simulink model "pmsm_drive"  (R2020b)
settings: Solver=VariableStepAuto  StartTime=0.0  StopTime=0.6  FixedStep=Ts  RelTol=1e-3  AbsTol=1e-3  EnableMultiTasking=on
PreLoadFcn:
  | % Control parameters
  | Ts = 2e-6;   % Fundamental sample time
  | fsw = 2e3;   % Switching frequency (Hz)
  | fc = fsw*10; % Control loop frequency (Hz)
  | Tsc = 1/fc;  % Control loop sample time
  | 
  | % PMSM parameters
  | PM = 0.03; % Permanent magnet flux linkage
  | Ld = 2e-4;  % d-axis inductance
  | Lq = 2e-4;  % q-axis inductance
  | L0 = 2e-4;  % 0-axis inductance
  | Rs = 0.013; % Stator resistance
  | N = 6; % Number of pole pairs
  | J = 0.2; % Moment of inertia
  | 
  | % Operating and derived limits
  | Imax = 100;  % Max stator current (peak value)
  | Tmax = 1.5*N*PM*Imax; % Max lectromagnetic torque
  | fnom = 100;  % Nominal frequency (Hz)
  | rpm_nom = 60*fnom/N;      % Nominal rotor speed (rpm)
  | omegam_nom = 2*pi*fnom/N; % Nominal mechanical rotor speed
  | Pmax = omegam_nom*Tmax;     % Maximum power
StopFcn:
  | ee_addSimlogTimeStamp(bdroot)
undefined symbols (not defined in the file or in its folder): ee_sli_rtmsupport, gcbh
libraries: fl_lib x10, nesl_utility x8, ee_lib x3, eeTransforms x2, eePmsmCurrentController x1, eePmsmCurrentReferenceGen x1, eeVelocityController x1, mcbplantlib x1
CloseFcn:
  | try,close(h1_ee_pmsm_drive),end
  | clear h1_ee_pmsm_drive
  | try,close(h2_ee_pmsm_drive),end
  | clear h2_ee_pmsm_drive
  | try,close(h3_ee_pmsm_drive),end
  | clear h3_ee_pmsm_drive
  | try,close(h4_ee_pmsm_drive),end
  | clear h4_ee_pmsm_drive
Description:
  | Three-Phase PMSM Drive
settings Model: Creator=The MathWorks, Inc.  LastModifiedBy=Student
settings SolverCC: AutoScaleAbsTol=off  MaxConsecutiveMinStep=2  ZeroCrossAlgorithm=Adaptive
settings DataIOCC: LimitDataPoints=on  MaxDataPoints=690000  SaveFormat=Array  ReturnWorkspaceOutputs=off  SignalLoggingName=logsout_ee_pmsm_drive
settings OptimizationCC: LifeSpan=inf
settings DebuggingCC: UnderspecifiedInitializationDetection=Classic  MergeDetectMultiDrivingBlocksExec=none  MaxConsecutiveZCsMsg=none  IgnoredZcDiagnostic=none  AllowSymbolicDim=off  PregeneratedLibrarySubsystemCodeDiagnostic=none  SFUnexpectedBacktrackingDiag=warning  SFNoUnconditionalDefaultTransitionDiag=warning  SFExecutionAtInitializationDiag=none  ArithmeticOperatorsInVariantConditions=warning
settings HardwareCC: ProdBitPerPointer=32  ProdBitPerSizeT=32  ProdBitPerPtrDiffT=32  ProdLargestAtomicFloat=None  ProdIntDivRoundTo=Undefined  ProdEndianess=Unspecified  ProdWordSize=32  ProdHWDeviceType=32-bit Generic
settings ModelReferenceCC: PropagateSignalLabelsOutOfModel=off
settings SFSimCC: SimUseLocalCustomCode=off
settings RTWCC: RTWUseLocalCustomCode=off
settings CodeAppCC: StateflowObjectComments=on
settings GRTTargetCC: TargetLangStandard=C89/C90 (ANSI)
settings ConfigComp: CovMetricSettings=dw  CovSaveCumulativeToWorkspaceVar=on  CovSaveSingleToWorkspaceVar=on  CovExternalEMLEnable=off  CovSFcnEnable=off
settings SimscapeCC: SimscapeLogType=all  SimscapeLogSimulationStatistics=on  SimscapeLogName=simlog_ee_pmsm_drive  SimscapeLogDataHistory=690000

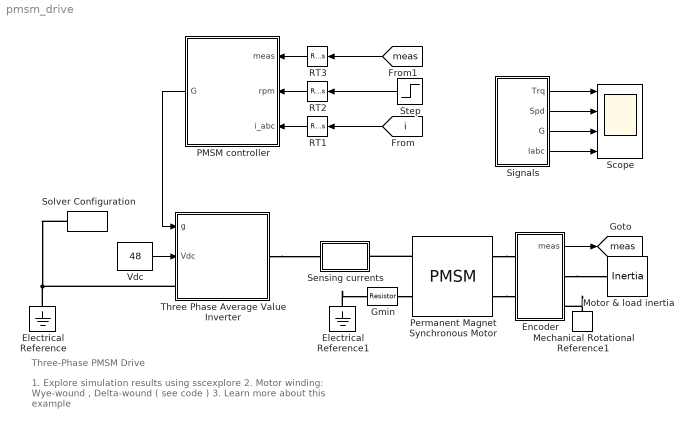
== system pmsm_drive ==
  note: Three-Phase PMSM Drive
  note: 1. Explore simulation results using sscexplore
      | 2. Motor winding: Wye-wound , Delta-wound ( see code )
      | 3. Learn more about this example
  Electrical Reference : fl_lib/Electrical/Electrical Elements/Electrical Reference
      settings: SourceProductName=Foundation Library
  Electrical Reference1 : fl_lib/Electrical/Electrical Elements/Electrical Reference
      settings: SourceProductName=Foundation Library
  Encoder : Subsystem
  Gmin : fl_lib/Electrical/Electrical Elements/Resistor  R=1e6 Ohm  i_specify=off  i_priority=High  i=0 A  i_nominal_specify=off  i_nominal_unit=A  i_nominal_value=1  v_specify=off  v_priority=High  v=0 V  v_nominal_specify=off  v_nominal_unit=V  v_nominal_value=1
      settings: SourceProductName=Foundation Library
  Mechanical Rotational Reference1 : fl_lib/Mechanical/Rotational Elements/Mechanical Rotational Reference
      settings: SourceProductName=Foundation Library
  Motor & load inertia : fl_lib/Mechanical/Rotational Elements/Inertia  inertia=J kg*m^2  num_ports=foundation.enum.numPorts2.one  w_specify=on  w_priority=High  w=0 rpm  w_nominal_specify=off  w_nominal_unit=rad/s  w_nominal_value=1  t_specify=off  t_priority=High  t=0 N*m  t_nominal_specify=off  t_nominal_unit=N*m  t_nominal_value=1
      settings: SourceProductName=Foundation Library
  PMSM controller : Subsystem
  Permanent Magnet Synchronous Motor : ee_lib/Electromechanical/Permanent Magnet/PMSM  winding_type=ee.enum.statorconnection.wye  machine_param=ee.enum.pmsm.parameterization.constant  nPolePairs=N  pmflux_param=ee.enum.pmflux.fluxlinkage  pm_flux_linkage=PM Wb  torque_constant=0.18 N*m/A  back_emf_constant=0.18 V/(rad/s)  stator_param=ee.enum.statorparam.LdLqL0  Ld=Ld H  Lq=Lq H  idVec=[-200, 0, 200] A  iqVec=[-200, 0, 200] A  LdMatrix=0.0002 * ones(3, 3) H  LqMatrix=0.0002 * ones(3, 3) H  PmMatrix=0.1 * ones(3, 3) Wb  ktMatrix=0.18 * ones(3, 3) N*m/A  keMatrix=0.18 * ones(3, 3) V/(rad/s)  L0=L0 H  Ls=0.0002 H  Lm=0.00002 H  Ms=0.00002 H  Rs=Rs Ohm  zero_sequence=ee.enum.park.zerosequence.exclude  J=0 kg*m^2  lam=0 N*m/(rad/s)  axes_param=ee.enum.rotorangle.qaxis  i_d_specify=off  i_d_priority=None  i_d=0 A  i_d_nominal_specify=off  i_d_nominal_unit=A  i_d_nominal_value=1  i_q_specify=off  i_q_priority=None  i_q=0 A  i_q_nominal_specify=off  i_q_nominal_unit=A  i_q_nominal_value=1  torque_specify=off  torque_priority=None  torque=0 N*m  torque_nominal_specify=off  torque_nominal_unit=N*m  torque_nominal_value=1  angular_velocity_specify=on  angular_velocity_priority=None  angular_velocity=0 rpm  angular_velocity_nominal_specify=off  angular_velocity_nominal_unit=rpm  angular_velocity_nominal_value=1  angular_position_specify=on  angular_position_priority=High  angular_position=0 rad  angular_position_nominal_specify=off  angular_position_nominal_unit=deg  angular_position_nominal_value=1  loss_param=ee.enum.ironloss.none  losses_oc=[0, 0, 0] W  losses_sc=[0, 0, 0] W  f_losses=60 Hz  Isc_losses=95 A  Tmeas=298.15 K  alpha=3.93e-3 1/K  alpha_flux=-0.001 1/K  stator_thermal_mass=100 J/K  rotor_thermal_mass=200 J/K  Rm_percent_rotor=90  Rd_percent_rotor=30  temperatureA_specify=off  temperatureA_priority=High  temperatureA=25 degC  temperatureA_nominal_specify=off  temperatureA_nominal_unit=degC  temperatureA_nominal_value=1  temperatureB_specify=off  temperatureB_priority=High  temperatureB=25 degC  temperatureB_nominal_specify=off  temperatureB_nominal_unit=degC  temperatureB_nominal_value=1  temperatureC_specify=off  temperatureC_priority=High  temperatureC=25 degC  temperatureC_nominal_specify=off  temperatureC_nominal_unit=degC  temperatureC_nominal_value=1  temperatureR_specify=off  temperatureR_priority=High  temperatureR=25 degC  temperatureR_nominal_specify=off  temperatureR_nominal_unit=degC  temperatureR_nominal_value=1
      settings: SourceProductName=Electrical  InternalSimscapePortConfiguration="{\"Bottom\":[],\"Left\":[{\"id\":\"N\",\"label\":\"~\",\"type\":\"foundation.electrical.three_phase\"},{\"id\":\"n\",\"label\":\"n\",\"type\":\"foundation.electrical.electrical\"}],\"Right\":[{\"id\":\"R\",\"label\":\"R\",\"type\":\"foundation.mechanical.rotational.rotational\"},{\"id\":\"C\",\"label\":\"C\",\"type\":\"foundation.mechanical.rotational.rotational\"}],\"Top\":[]}"
  RT1 : RateTransition  OutPortSampleTime=Tsc
  RT2 : RateTransition  OutPortSampleTime=Tsc
  RT3 : RateTransition  OutPortSampleTime=Tsc
  Scope : Scope  NumInputPorts=4
  Sensing currents : Subsystem
      mask Display: disp('i')
  "Signals " : Subsystem
  Solver Configuration : nesl_utility/Solver Configuration  PhysicalDomain=network_engine_domain  SubClassName=solver  LeftPortType=input  RightPortType=generic  Tones=[]  Harmonics=[]  SimulateNoise=off  Profile=off  UseLocalSampling=off  EnableSwitchedLinearOptims=on  FrequencyDomain=off  UseCCode=off  RelTol=0.001  AbsTol=1e-06  MinStep=1e-09  ToWorkspace=off  RevertToSquareIcSolve=off  NumHomotopyIterations=100  PhasorMode=off  PhasorModeNumHarmonics=1  DoDC=off  ResidualTolerance=1e-9  UseLocalSolver=off  LocalSolverChoice=NE_BACKWARD_EULER_ADVANCER  LocalSolverSampleTime=Ts  DoFixedCost=off  MaxNonlinIter=4  MaxModeIter=2  ComputeImpulses=off  ImpulseIterations=2  LinearAlgebra=auto  EquationFormulation=NE_TIME_EF  DelaysMemoryBudget=1024  AutomaticFiltering=on  FilteringTimeConstant=0.001  PartitionStorageMethod=AS_NEEDED  PartitionMemoryBudget=1024  PartitionMethod=FAST
      settings: SourceProductName=Utilities
  Step : Step  Time=0.1  After=500  SampleTime=0
  Three Phase Average Value Inverter : Subsystem
  Vdc : Constant  Value=48  SampleTime=Tsc
  tag scope: meas=global
  wires:
  Step/1 -> RT2/1
  RT3/1 -> PMSM controller/1(meas)
  RT2/1 -> PMSM controller/2(rpm)
  RT1/1 -> PMSM controller/3(i_abc)
  "Signals "/2(Spd) -> Scope/2
  "Signals "/4(Iabc) -> Scope/4
  "Signals "/3(G) -> Scope/3
  "Signals "/1(Trq) -> Scope/1
  [i] -> RT1/1
  Encoder/1(meas) -> [meas]
  [meas] -> RT3/1
  Vdc/1 -> Three Phase Average Value Inverter/2(Vdc)
  PMSM controller/1(G) -> Three Phase Average Value Inverter/1(g)
  connections:
  Permanent Magnet Synchronous Motor/RConn1 -- Encoder/LConn1
  Permanent Magnet Synchronous Motor/RConn2 -- Encoder/LConn2
  Encoder/RConn1 -- Motor & load inertia/LConn1
  Mechanical Rotational Reference1/LConn1 -- Encoder/RConn2
  Electrical Reference/LConn1 -- Three Phase Average Value Inverter/LConn1 -- Solver Configuration/RConn1
  Electrical Reference1/LConn1 -- Gmin/LConn1
  Three Phase Average Value Inverter/RConn1 -- Sensing currents/LConn1
  Permanent Magnet Synchronous Motor/LConn1 -- Sensing currents/RConn1
  Gmin/RConn1 -- Permanent Magnet Synchronous Motor/LConn2

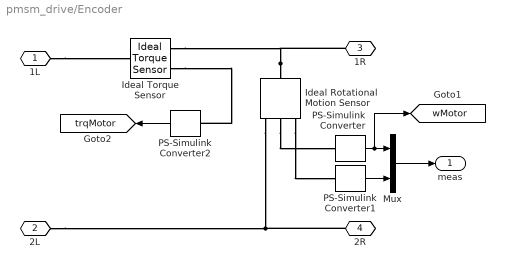
== system pmsm_drive/Encoder ==
  Ideal Rotational Motion Sensor : fl_lib/Mechanical/Mechanical Sensors/Ideal Rotational Motion Sensor  wrap_angle=simscape.enum.onoff.off  offset=0 deg
      settings: SourceProductName=Foundation Library
  Ideal Torque Sensor : fl_lib/Mechanical/Mechanical Sensors/Ideal Torque Sensor
      settings: SourceProductName=Foundation Library
  Mux : Mux  Inputs=2
  PS-Simulink Converter : nesl_utility/PS-Simulink Converter  PhysicalDomain=network_engine_domain  SubClassName=ps_output  LeftPortType=input  RightPortType=output  PseudoPeriodic=off  Frequencies=[]  Unit=rad/s  AffineConversion=off
      settings: SourceProductName=Utilities
  PS-Simulink Converter1 : nesl_utility/PS-Simulink Converter  PhysicalDomain=network_engine_domain  SubClassName=ps_output  LeftPortType=input  RightPortType=output  PseudoPeriodic=off  Frequencies=[]  Unit=rad  AffineConversion=off
      settings: SourceProductName=Utilities
  PS-Simulink Converter2 : nesl_utility/PS-Simulink Converter  PhysicalDomain=network_engine_domain  SubClassName=ps_output  LeftPortType=input  RightPortType=output  PseudoPeriodic=off  Frequencies=[]  Unit=N*m  AffineConversion=off
      settings: SourceProductName=Utilities
  1L : PMIOPort  Side=Left
  2L : PMIOPort  Port=2  Side=Left
  1R : PMIOPort  Port=3  Side=Right
  2R : PMIOPort  Port=4  Side=Right
  meas : Outport  VectorParamsAs1DForOutWhenUnconnected=off
  tag scope: trqMotor=global, wMotor=global
  wires:
  PS-Simulink Converter2/1 -> [trqMotor]
  Mux/1 -> meas/1
  PS-Simulink Converter1/1 -> Mux/2
  PS-Simulink Converter/1 -> [wMotor], Mux/1
  connections:
  Ideal Torque Sensor/RConn2 -- PS-Simulink Converter2/LConn1
  1L/RConn1 -- Ideal Torque Sensor/LConn1
  2R/RConn1 -- 2L/RConn1 -- Ideal Rotational Motion Sensor/RConn1
  Ideal Rotational Motion Sensor/LConn1 -- 1R/RConn1 -- Ideal Torque Sensor/RConn1
  Ideal Rotational Motion Sensor/RConn2 -- PS-Simulink Converter/LConn1
  Ideal Rotational Motion Sensor/RConn3 -- PS-Simulink Converter1/LConn1

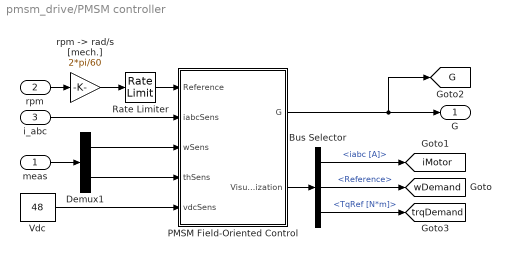
== system pmsm_drive/PMSM controller ==
  meas : Inport
  rpm : Inport  Port=2
  i_abc : Inport  Port=3
  Bus Selector : BusSelector  OutputSignals=iabc [A],Reference,TqRef [N*m]
  Demux1 : Demux  Outputs=2
  PMSM Field-Oriented Control : Subsystem  AncestorBlock=eePmsmFieldOrientedControl/PMSM Field-Oriented Control  LoadFcn=ee_sli_rtmsupport( 'loadfcn', gcbh );  mask(PMSM Field-Oriented Control){winding_type=Wye-wound, CtrlMode=Velocity control, Vnom=48, Pmax=Pmax, Tmax=Tmax*1.5, p=N, Vdc_on=10, Ts=Ts, Tsc=Tsc, CtrlType=PI control, Kp_w=60, Ki_w=300*2, Kv_w=1, Kaw_w=1000, RefType=Zero d-axis control, rpmVec=[0, 3000], TqVec=[-100, 0, 100], VdcVec=[300, 350], PWMMode=SPWM: sinusoidal PWM, ModFactor=1, idMatrix=zeros(2,3,2), iqMatrix=zeros(2,3,2), psim=PM, Ld=0.00024, Lq=0.00029, Rs=0.01, AxisAlignment=Q-axis, Kp_id=0.1, Ki_id=10, Kaw_id=1000, Kp_iq=0.1, Ki_iq=10, Kaw_iq=1000, AxisPrio=Q-axis, ActZC=off, ActFF=on, ParamTypeFF=Constant parameters, LdFF=Ld, LqFF=Lq, psimFF=PM, idVect=[-200, 0, 200], iqVect=[-200, 0, 200], LdMatrix=0.0002 * ones(3, 3), LqMatrix=0.0002 * ones(3, 3), psimMatrix=0.04 * ones(3, 3), CPWMMode=SPWM: sinusoidal PWM, SamplingMode=Natural, fsw=fsw}
      mask prompts: winding_type "physmod:ee:library:comments:control:eePmsmFieldOrientedControl:WindingType_MP"; CtrlMode "physmod:ee:library:comments:control:eePmsmFieldOrientedControl:ControlMode_MP"; Vnom "physmod:ee:library:comments:control:eePmsmFieldOrientedControl:NominalDclinkVoltageV_MP"; Pmax "physmod:ee:library:comments:control:eePmsmFieldOrientedControl:MaximumPowerW_MP"; Tmax "physmod:ee:library:comments:control:eePmsmFieldOrientedControl:MaximumTorqueNm_MP"; p "physmod:ee:library:comments:control:eePmsmFieldOrientedControl:NumberOfRotorPolePairs_MP"; Vdc_on "physmod:ee:library:comments:control:eePmsmFieldOrientedControl:InverterDclinkVoltageThresholdV_MP"; Ts "physmod:ee:library:comments:control:eePmsmFieldOrientedControl:FundamentalSampleTimes_MP"; Tsc "physmod:ee:library:comments:control:eePmsmFieldOrientedControl:ControlSampleTimes_MP"; CtrlType "physmod:ee:library:comments:control:eePmsmFieldOrientedControl:ControlType_MP"; Kp_w "physmod:ee:library:comments:control:eePmsmFieldOrientedControl:ControllerProportionalGain_MP"; Ki_w "physmod:ee:library:comments:control:eePmsmFieldOrientedControl:ControllerIntegralGain_MP"; Kv_w "physmod:ee:library:comments:control:eePmsmFieldOrientedControl:PControllerProportionalGain_MP"; Kaw_w "physmod:ee:library:comments:control:eePmsmFieldOrientedControl:IntegralAntiwindupGain_MP"; RefType "physmod:ee:library:comments:control:eePmsmFieldOrientedControl:CurrentReferences_MP"; rpmVec "physmod:ee:library:comments:control:eePmsmFieldOrientedControl:MechanicalSpeedVectorWMechanicalrpm_MP"; TqVec "physmod:ee:library:comments:control:eePmsmFieldOrientedControl:TorqueReferenceVectorTqRefNm_MP"; VdcVec "physmod:ee:library:comments:control:eePmsmFieldOrientedControl:DClinkVoltageVectorVdcV_MP"; PWMMode "physmod:ee:library:comments:control:eePmsmCurrentReferenceGen:PWMMethod_MP"; ModFactor "physmod:ee:library:comments:control:eePmsmCurrentReferenceGen:ModulationFactor_MP"; idMatrix "physmod:ee:library:comments:control:eePmsmFieldOrientedControl:DaxisCurrentReferenceMatrixIdwMechanicalTqRefVdcA_MP"; iqMatrix "physmod:ee:library:comments:control:eePmsmFieldOrientedControl:QaxisCurrentReferenceMatrixIqwMechanicalTqRefVdcA_MP"; psim "physmod:ee:library:comments:control:eePmsmFieldOrientedControl:PermanentMagnetFluxLinkageWb_MP"; Ld "physmod:ee:library:comments:control:eePmsmFieldOrientedControl:DaxisInductanceH_MP"; Lq "physmod:ee:library:comments:control:eePmsmFieldOrientedControl:QaxisInductanceH_MP"; Rs "physmod:ee:library:comments:control:eePmsmFieldOrientedControl:StatorResistanceOhm_MP"; AxisAlignment "physmod:ee:library:comments:control:eePmsmFieldOrientedControl:PhaseaAxisAlignment_MP"; Kp_id "physmod:ee:library:comments:control:eePmsmFieldOrientedControl:DaxisCurrentProportionalGain_MP"; Ki_id "physmod:ee:library:comments:control:eePmsmFieldOrientedControl:DaxisCurrentIntegralGain_MP"; Kaw_id "physmod:ee:library:comments:control:eePmsmFieldOrientedControl:DaxisCurrentAntiwindupGain_MP"; Kp_iq "physmod:ee:library:comments:control:eePmsmFieldOrientedControl:QaxisCurrentProportionalGain_MP"; Ki_iq "physmod:ee:library:comments:control:eePmsmFieldOrientedControl:QaxisCurrentIntegralGain_MP"; Kaw_iq "physmod:ee:library:comments:control:eePmsmFieldOrientedControl:QaxisCurrentAntiwindupGain_MP"; AxisPrio "physmod:ee:library:comments:control:eePmsmFieldOrientedControl:AxisPrioritization_MP"; ActZC "physmod:ee:library:comments:control:eePmsmFieldOrientedControl:EnableZeroCancellation_MP"; ActFF "physmod:ee:library:comments:control:eePmsmFieldOrientedControl:EnablePrecontrolVoltage_MP"; ParamTypeFF "physmod:ee:library:comments:control:eePmsmFieldOrientedControl:MachineParameters_MP"; LdFF "physmod:ee:library:comments:control:eePmsmFieldOrientedControl:DaxisInductanceForFeedforwardPrecontrolH_MP"; LqFF "physmod:ee:library:comments:control:eePmsmFieldOrientedControl:QaxisInductanceForFeedforwardPrecontrolH_MP"; psimFF "physmod:ee:library:comments:control:eePmsmFieldOrientedControl:PermanentMagnetFluxLinkageForFeedforwardPrecontrolWb_MP"; idVect "physmod:ee:library:comments:control:eePmsmFieldOrientedControl:DaxisCurrentVectorIdA_MP"; iqVect "physmod:ee:library:comments:control:eePmsmFieldOrientedControl:QaxisCurrentVectorIqA_MP"; LdMatrix "physmod:ee:library:comments:control:eePmsmFieldOrientedControl:LdMatrixLdidiqH_MP"; LqMatrix "physmod:ee:library:comments:control:eePmsmFieldOrientedControl:LqMatrixLqidiqH_MP"; psimMatrix "physmod:ee:library:comments:control:eePmsmFieldOrientedControl:PermanentMagnetFluxLinkageMatrixPMidiqWb_MP"; CPWMMode "physmod:ee:library:comments:control:eePmsmFieldOrientedControl:PWMMethod_MP"; SamplingMode "physmod:ee:library:comments:control:eePmsmFieldOrientedControl:SamplingMode_MP"; fsw "physmod:ee:library:comments:control:eePmsmFieldOrientedControl:SwitchingFrequencyHz_MP"
      mask help: physmod:ee:library:comments:control:eePmsmFieldOrientedControl:PMSMFieldOrientedControl_MD
      mask init:
      | if ParamTypeFF == 1
      |     idVect = [-200, 200];
      |     iqVect = [-200, 200];
      |     LdMatrix = LdFF*ones(2, 2);
      |     LqMatrix = LqFF*ones(2, 2);
      |     psimMatrix = psimFF*ones(2, 2);
      | end
      | 
      | switch winding_type
      |     case 1
      |         theta_offset = 0;
      |     case 2
      |         theta_offset = -(120/p)*pi/180;
      |     otherwise
      |         theta_offset = 0;
      | end
      | 
      | switch CPWMMode
      |     case 'SPWM: sinusoidal PWM'
      |         set_param(gcb,'PWMMode','SPWM: sinusoidal PWM');
      |     case 'SVM: space vector modulation'
      |         set_param(gcb,'PWMMode','SVM: space vector modulation')
      | end
      settings: CopyFcn=ee_sli_rtmsupport( 'copyfcn', gcbh );  DeleteFcn=ee_sli_rtmsupport( 'deletefcn', gcbh );  ModelCloseFcn=ee_sli_rtmsupport( 'modelclosefcn', gcbh );  PostSaveFcn=ee_sli_rtmsupport( 'postsavefcn', gcbh );  PreCopyFcn=ee_sli_rtmsupport( 'precopyfcn', gcbh );  OpenFcn=ee_sli_rtmsupport( 'openfcn', gcbh );  CloseFcn=ee_sli_rtmsupport( 'closefcn', gcbh );  PreDeleteFcn=ee_sli_rtmsupport( 'predeletefcn', gcbh );
      mask Help: web(nesl_help(gcbh))
      mask TypeOptions winding_type: physmod:ee:library:comments:control:eePmsmFieldOrientedControl:WyeWound_PV | physmod:ee:library:comments:control:eePmsmFieldOrientedControl:DeltaWound_PV
      mask Callback winding_type: ee.mask.callbackPopupPmsmFoc(gcb);
      mask TypeOptions CtrlMode: physmod:ee:library:comments:control:eePmsmFieldOrientedControl:VelocityControl_PV | physmod:ee:library:comments:control:eePmsmFieldOrientedControl:TorqueControl_PV
      mask Callback CtrlMode: ee.mask.callbackPopupPmsmFoc(gcb);
      mask TypeOptions Vnom:
      | Outer loop control/PMSM Current Reference
      | Generator/Vnom
      mask TypeOptions Pmax:
      | Outer loop control/PMSM Current Reference
      | Generator/Pmax
      mask TypeOptions Tmax:
      | Outer loop control/PMSM Current Reference
      | Generator/Tmax
      mask TypeOptions CtrlType: Outer loop control/Velocity Controller/CtrlType
      mask Callback CtrlType: ee.mask.callbackPopupPmsmFoc(gcb);
      mask TypeOptions Kp_w: Outer loop control/Velocity Controller/Kp_w
      mask TypeOptions Ki_w: Outer loop control/Velocity Controller/Ki_w
      mask TypeOptions Kv_w: Outer loop control/Velocity Controller/Kv_w
      mask TypeOptions Kaw_w: Outer loop control/Velocity Controller/Kaw_w
      mask TypeOptions RefType:
      | Outer loop control/PMSM Current Reference
      | Generator/RefType
      mask Callback RefType: ee.mask.callbackPopupPmsmFoc(gcb);
      mask TypeOptions rpmVec:
      | Outer loop control/PMSM Current Reference
      | Generator/rpmVec
      mask TypeOptions TqVec:
      | Outer loop control/PMSM Current Reference
      | Generator/TqVec
      mask TypeOptions VdcVec:
      | Outer loop control/PMSM Current Reference
      | Generator/VdcVec
      mask TypeOptions PWMMode:
      | Outer loop control/PMSM Current Reference
      | Generator/PWMMode
      mask TypeOptions ModFactor:
      | Outer loop control/PMSM Current Reference
      | Generator/ModFactor
      mask TypeOptions idMatrix:
      | Outer loop control/PMSM Current Reference
      | Generator/idMatrix
      mask TypeOptions iqMatrix:
      | Outer loop control/PMSM Current Reference
      | Generator/iqMatrix
      mask TypeOptions psim:
      | Outer loop control/PMSM Current Reference
      | Generator/psim
      mask TypeOptions Ld:
      | Outer loop control/PMSM Current Reference
      | Generator/Ld
      mask TypeOptions Lq:
      | Outer loop control/PMSM Current Reference
      | Generator/Lq
      mask TypeOptions Rs:
      | Outer loop control/PMSM Current Reference
      | Generator/Rs
      mask TypeOptions AxisAlignment: Inner loop control/Park Transform/AxisAlignment
      mask TypeOptions Kp_id:
      | Inner loop control/PMSM Current Controller
      | with Pre-Control/Kp_id
      mask TypeOptions Ki_id:
      | Inner loop control/PMSM Current Controller
      | with Pre-Control/Ki_id
      mask TypeOptions Kaw_id:
      | Inner loop control/PMSM Current Controller
      | with Pre-Control/Kaw_id
      mask TypeOptions Kp_iq:
      | Inner loop control/PMSM Current Controller
      | with Pre-Control/Kp_iq
      mask TypeOptions Ki_iq:
      | Inner loop control/PMSM Current Controller
      | with Pre-Control/Ki_iq
      mask TypeOptions Kaw_iq:
      | Inner loop control/PMSM Current Controller
      | with Pre-Control/Kaw_iq
      mask TypeOptions AxisPrio:
      | Inner loop control/PMSM Current Controller
      | with Pre-Control/AxisPrio
      mask TypeOptions ActZC:
      | Inner loop control/PMSM Current Controller
      | with Pre-Control/ActZC
      mask TypeOptions ActFF:
      | Inner loop control/PMSM Current Controller
      | with Pre-Control/ActFF
      mask Callback ActFF: ee.mask.callbackPopupPmsmFoc(gcb);
      mask TypeOptions ParamTypeFF: physmod:ee:library:comments:control:eePmsmFieldOrientedControl:ConstantParameters_PV | physmod:ee:library:comments:control:eePmsmFieldOrientedControl:LookupTableBasedParameters_PV
      mask Callback ParamTypeFF: ee.mask.callbackPopupPmsmFoc(gcb);
      mask TypeOptions idVect:
      | Inner loop control/PMSM Current Controller
      | with Pre-Control/idVect
      mask TypeOptions iqVect:
      | Inner loop control/PMSM Current Controller
      | with Pre-Control/iqVect
      mask TypeOptions LdMatrix:
      | Inner loop control/PMSM Current Controller
      | with Pre-Control/LdMatrix
      mask TypeOptions LqMatrix:
      | Inner loop control/PMSM Current Controller
      | with Pre-Control/LqMatrix
      mask TypeOptions psimMatrix:
      | Inner loop control/PMSM Current Controller
      | with Pre-Control/psimMatrix
      mask TypeOptions CPWMMode:
      | PWM/PWM Generator
      | (Three-phase, Two-level)/CPWMMode
      mask TypeOptions SamplingMode:
      | PWM/PWM Generator
      | (Three-phase, Two-level)/SamplingMode
      mask DialogControl Container4 Prompt: physmod:ee:library:comments:control:eePmsmFieldOrientedControl:tab_General
      mask DialogControl winding_type Prompt: Winding type
      mask DialogControl CtrlMode Prompt: Control mode
      mask DialogControl Vnom Prompt: Nominal dc-link voltage (V)
      mask DialogControl Pmax Prompt: Maximum power (W)
      mask DialogControl Tmax Prompt: Maximum torque (N*m)
      mask DialogControl p Prompt: Number of rotor pole pairs
      mask DialogControl Vdc_on Prompt: Inverter dc-link voltage threshold (V)
      mask DialogControl Ts Prompt: Fundamental sample time (s)
      mask DialogControl Tsc Prompt: Control sample time (s)
      mask DialogControl Container7 Prompt: physmod:ee:library:comments:control:eePmsmFieldOrientedControl:tab_OuterLoop
      mask DialogControl CtrlType Prompt: Control type
      mask DialogControl Kp_w Prompt: Controller proportional gain
      mask DialogControl Ki_w Prompt: Controller integral gain
      mask DialogControl Kv_w Prompt: P controller proportional gain
      mask DialogControl Kaw_w Prompt: Integral anti-windup gain
      mask DialogControl RefType Prompt: Current references
      mask DialogControl rpmVec Prompt: Mechanical speed vector, wMechanical (rpm)
      mask DialogControl TqVec Prompt: Torque reference vector, TqRef (N*m)
      mask DialogControl VdcVec Prompt: DC-link voltage vector, Vdc (V)
      mask DialogControl PWMMode Prompt: PWM method
      mask DialogControl ModFactor Prompt: Modulation factor
      mask DialogControl idMatrix Prompt: D-axis current reference matrix, id(wMechanical,TqRef,Vdc), (A)
      mask DialogControl iqMatrix Prompt: Q-axis current reference matrix, iq(wMechanical,TqRef,Vdc), (A)
      mask DialogControl psim Prompt: Permanent magnet flux linkage (Wb)
      mask DialogControl Ld Prompt: D-axis inductance (H)
      mask DialogControl Lq Prompt: Q-axis inductance (H)
      mask DialogControl Rs Prompt: Stator resistance (Ohm)
      mask DialogControl Container8 Prompt: physmod:ee:library:comments:control:eePmsmFieldOrientedControl:tab_InnerLoop
      mask DialogControl AxisAlignment Prompt: Phase-a axis alignment
      mask DialogControl Kp_id Prompt: D-axis current proportional gain
      mask DialogControl Ki_id Prompt: D-axis current integral gain
      mask DialogControl Kaw_id Prompt: D-axis current anti-windup gain
      mask DialogControl Kp_iq Prompt: Q-axis current proportional gain
      mask DialogControl Ki_iq Prompt: Q-axis current integral gain
      mask DialogControl Kaw_iq Prompt: Q-axis current anti-windup gain
      mask DialogControl AxisPrio Prompt: Axis prioritization
      mask DialogControl ActZC Prompt: Enable zero cancellation
      mask DialogControl ActFF Prompt: Enable pre-control voltage
      mask DialogControl ParamTypeFF Prompt: Machine parameters
      mask DialogControl LdFF Prompt: D-axis inductance for feed-forward pre-control (H)
      mask DialogControl LqFF Prompt: Q-axis inductance for feed-forward pre-control (H)
      mask DialogControl psimFF Prompt: Permanent magnet flux linkage for feed-forward pre-control (Wb)
      mask DialogControl idVect Prompt: D-axis current vector, id (A)
      mask DialogControl iqVect Prompt: Q-axis current vector, iq (A)
      mask DialogControl LdMatrix Prompt: Ld matrix, Ld(id,iq), (H)
      mask DialogControl LqMatrix Prompt: Lq matrix, Lq(id,iq), (H)
      mask DialogControl psimMatrix Prompt: Permanent magnet flux linkage matrix, PM(id,iq), (Wb)
      mask DialogControl Container9 Prompt: physmod:ee:library:comments:control:eePmsmFieldOrientedControl:tab_PWM
      mask DialogControl CPWMMode Prompt: PWM method
      mask DialogControl SamplingMode Prompt: Sampling mode
      mask DialogControl fsw Prompt: Switching frequency (Hz)
  Rate Limiter : RateLimiter  RisingSlewLimit=Tmax/J  FallingSlewLimit=-Tmax/J  SampleTimeMode=inherited
  Vdc : Constant  Value=48  SampleTime=Tsc
  "rpm -> rad/s [mech.]" : Gain  Gain=2*pi/60
  G : Outport  VectorParamsAs1DForOutWhenUnconnected=off
  tag scope: G=global, iMotor=global, trqDemand=global, wDemand=global
  wires:
  PMSM Field-Oriented Control/1(G) -> G/1, [G]
  Vdc/1 -> PMSM Field-Oriented Control/5(vdcSens)
  PMSM Field-Oriented Control/2(Visualization) -> Bus Selector/1
  i_abc/1 -> PMSM Field-Oriented Control/2(iabcSens)
  meas/1 -> Demux1/1
  Demux1/1 -> PMSM Field-Oriented Control/3(wSens)
  Demux1/2 -> PMSM Field-Oriented Control/4(thSens)
  Bus Selector/1 -> [iMotor]  "<iabc [A]>"
  Bus Selector/2 -> [wDemand]  "<Reference>"
  Bus Selector/3 -> [trqDemand]  "<TqRef [N*m]>"
  rpm/1 -> "rpm -> rad/s [mech.]"/1
  Rate Limiter/1 -> PMSM Field-Oriented Control/1(Reference)
  "rpm -> rad/s [mech.]"/1 -> Rate Limiter/1

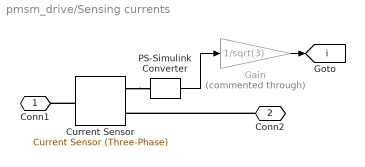
== system pmsm_drive/Sensing currents ==
  Current Sensor : ee_lib/Sensors & Transducers/Current Sensor (Three-Phase)
      settings: SourceProductName=Electrical
  Gain : Gain  Commented=through  Gain=1/sqrt(3)
  PS-Simulink Converter : nesl_utility/PS-Simulink Converter  PhysicalDomain=network_engine_domain  SubClassName=ps_output  LeftPortType=input  RightPortType=output  PseudoPeriodic=off  Frequencies=[]  Unit=A  AffineConversion=off
      settings: SourceProductName=Utilities
  Conn1 : PMIOPort  Side=Left
  Conn2 : PMIOPort  Port=2  Side=Right
  tag scope: i=global
  wires:
  PS-Simulink Converter/1 -> Gain/1
  Gain/1 -> [i]
  connections:
  Current Sensor/RConn1 -- PS-Simulink Converter/LConn1
  Conn2/RConn1 -- Current Sensor/RConn2
  Current Sensor/LConn1 -- Conn1/RConn1

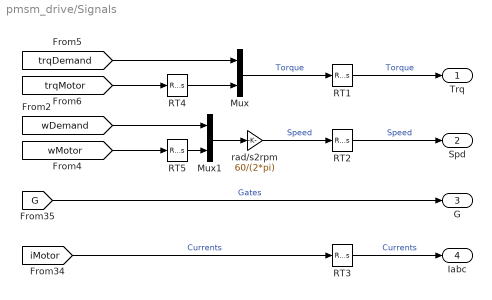
== system pmsm_drive/Signals  ==
  Mux : Mux  Inputs=2
  Mux1 : Mux  Inputs=2
  RT1 : RateTransition  OutPortSampleTime=Ts
  RT2 : RateTransition  OutPortSampleTime=Ts
  RT3 : RateTransition  OutPortSampleTime=Ts
  RT4 : RateTransition  OutPortSampleTime=Tsc
  RT5 : RateTransition  OutPortSampleTime=Tsc
  rad/s2rpm : Gain  Gain=60/(2*pi)
  Trq : Outport  VectorParamsAs1DForOutWhenUnconnected=off
  Spd : Outport  Port=2  VectorParamsAs1DForOutWhenUnconnected=off
  G : Outport  Port=3  VectorParamsAs1DForOutWhenUnconnected=off
  Iabc : Outport  Port=4  VectorParamsAs1DForOutWhenUnconnected=off
  wires:
  [trqDemand] -> Mux/1
  [G] -> G/1  "Gates"
  Mux1/1 -> rad/s2rpm/1
  Mux/1 -> RT1/1  "Torque"
  [iMotor] -> RT3/1  "Currents"
  [wDemand] -> Mux1/1
  rad/s2rpm/1 -> RT2/1  "Speed"
  [trqMotor] -> RT4/1
  [wMotor] -> RT5/1
  RT1/1 -> Trq/1  "Torque"
  RT2/1 -> Spd/1  "Speed"
  RT3/1 -> Iabc/1  "Currents"
  RT4/1 -> Mux/2
  RT5/1 -> Mux1/2

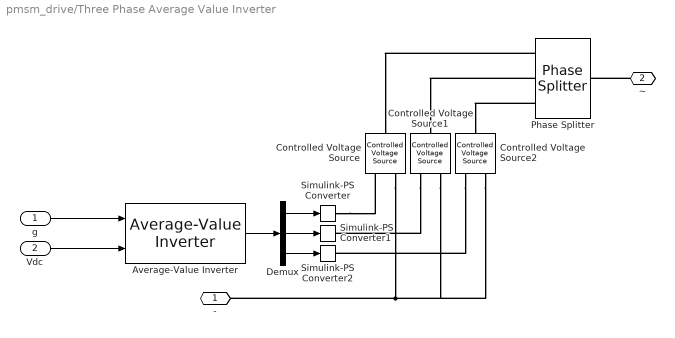
== system pmsm_drive/Three Phase Average Value Inverter ==
  g : Inport
  Vdc : Inport  Port=2
  Average-Value Inverter : mcbplantlib/Average-Value Inverter
  Controlled Voltage Source : fl_lib/Electrical/Electrical Sources/Controlled Voltage Source
  Controlled Voltage Source1 : fl_lib/Electrical/Electrical Sources/Controlled Voltage Source
  Controlled Voltage Source2 : fl_lib/Electrical/Electrical Sources/Controlled Voltage Source
  Demux : Demux  Outputs=3
  Phase Splitter : ee_lib/Connectors & References/Phase Splitter
      settings: SourceProductBaseCode=PS
  Simulink-PS Converter : nesl_utility/Simulink-PS Converter  PhysicalDomain=network_engine_domain  SubClassName=ps_input  LeftPortType=input  RightPortType=output  PseudoPeriodic=off  Frequencies=[]  NoiseDistribution=none  NoiseParameters=[]  Unit=1  AffineConversion=off  FilteringAndDerivatives=provide  SimscapeFilterOrder=1  InputFilterTimeConstant=0.001  UdotUserProvided=0
  Simulink-PS Converter1 : nesl_utility/Simulink-PS Converter  PhysicalDomain=network_engine_domain  SubClassName=ps_input  LeftPortType=input  RightPortType=output  PseudoPeriodic=off  Frequencies=[]  NoiseDistribution=none  NoiseParameters=[]  Unit=1  AffineConversion=off  FilteringAndDerivatives=provide  SimscapeFilterOrder=1  InputFilterTimeConstant=0.001  UdotUserProvided=0
  Simulink-PS Converter2 : nesl_utility/Simulink-PS Converter  PhysicalDomain=network_engine_domain  SubClassName=ps_input  LeftPortType=input  RightPortType=output  PseudoPeriodic=off  Frequencies=[]  NoiseDistribution=none  NoiseParameters=[]  Unit=1  AffineConversion=off  FilteringAndDerivatives=provide  SimscapeFilterOrder=1  InputFilterTimeConstant=0.001  UdotUserProvided=0
  - : PMIOPort  Tag=PMCPort  Side=Left
  ~ : PMIOPort  Tag=PMCPort  Port=2  Side=Right
  wires:
  Demux/3 -> Simulink-PS Converter2/1
  Vdc/1 -> Average-Value Inverter/2
  Demux/2 -> Simulink-PS Converter1/1
  Average-Value Inverter/1 -> Demux/1
  Demux/1 -> Simulink-PS Converter/1
  g/1 -> Average-Value Inverter/1
  connections:
  ~/RConn1 -- Phase Splitter/LConn1
  Controlled Voltage Source/RConn2 -- -/RConn1 -- Controlled Voltage Source1/RConn2 -- Controlled Voltage Source2/RConn2
  Simulink-PS Converter/RConn1 -- Controlled Voltage Source/RConn1
  Controlled Voltage Source2/RConn1 -- Simulink-PS Converter2/RConn1
  Phase Splitter/RConn3 -- Controlled Voltage Source2/LConn1
  Phase Splitter/RConn1 -- Controlled Voltage Source/LConn1
  Phase Splitter/RConn2 -- Controlled Voltage Source1/LConn1
  Controlled Voltage Source1/RConn1 -- Simulink-PS Converter1/RConn1

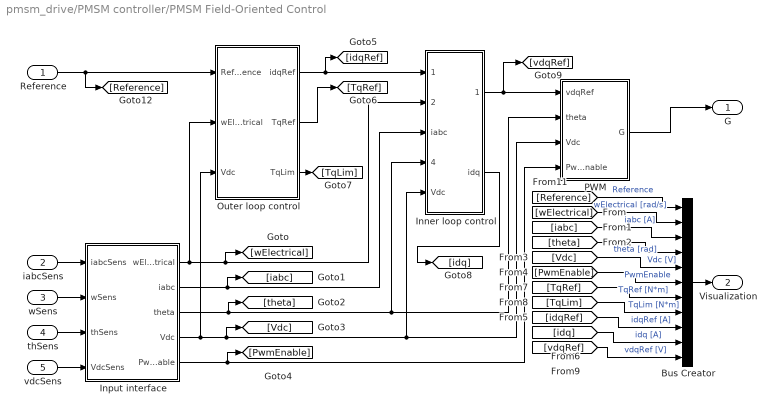
== system pmsm_drive/PMSM controller/PMSM Field-Oriented Control ==
  Reference : Inport  SampleTime=Tsc
  iabcSens : Inport  Port=2  SampleTime=Tsc
  wSens : Inport  Port=3  SampleTime=Tsc
  thSens : Inport  Port=4  SampleTime=Tsc
  vdcSens : Inport  Port=5  SampleTime=Tsc
  Bus Creator : BusCreator  Inputs=11
  Inner loop control : Subsystem
  Input interface : Subsystem
  Outer loop control : Subsystem
  PWM : Subsystem
  G : Outport  VectorParamsAs1DForOutWhenUnconnected=off
  Visualization : Outport  Port=2  VectorParamsAs1DForOutWhenUnconnected=off
  wires:
  [vdqRef] -> Bus Creator/11  "vdqRef [V]"
  [idq] -> Bus Creator/10  "idq [A]"
  [idqRef] -> Bus Creator/9  "idqRef [A]"
  [TqLim] -> Bus Creator/8  "TqLim [N*m]"
  [TqRef] -> Bus Creator/7  "TqRef [N*m]"
  [PwmEnable] -> Bus Creator/6  "PwmEnable"
  [Vdc] -> Bus Creator/5  "Vdc [V]"
  [theta] -> Bus Creator/4  "theta [rad]"
  [iabc] -> Bus Creator/3  "iabc [A]"
  [wElectrical] -> Bus Creator/2  "wElectrical [rad/s]"
  [Reference] -> Bus Creator/1  "Reference"
  Inner loop control/2(idq) -> [idq]
  Outer loop control/3(TqLim) -> [TqLim]
  Outer loop control/2(TqRef) -> [TqRef]
  Bus Creator/1 -> Visualization/1
  PWM/1(G) -> G/1
  Input interface/5(PwmEnable) -> PWM/4(PwmEnable), [PwmEnable]
  Inner loop control/1(vdqRef) -> PWM/1(vdqRef), [vdqRef]
  Input interface/1(wElectrical) -> Outer loop control/2(wElectrical), Inner loop control/2(wElectrical), [wElectrical]
  Input interface/4(Vdc) -> Outer loop control/3(Vdc), Inner loop control/5(Vdc), PWM/3(Vdc), [Vdc]
  Reference/1 -> Outer loop control/1(Reference), [Reference]
  vdcSens/1 -> Input interface/4(VdcSens)
  thSens/1 -> Input interface/3(thSens)
  wSens/1 -> Input interface/2(wSens)
  iabcSens/1 -> Input interface/1(iabcSens)
  Outer loop control/1(idqRef) -> Inner loop control/1(idq_ref), [idqRef]
  Input interface/3(theta) -> Inner loop control/4(theta), PWM/2(theta), [theta]
  Input interface/2(iabc) -> Inner loop control/3(iabc), [iabc]

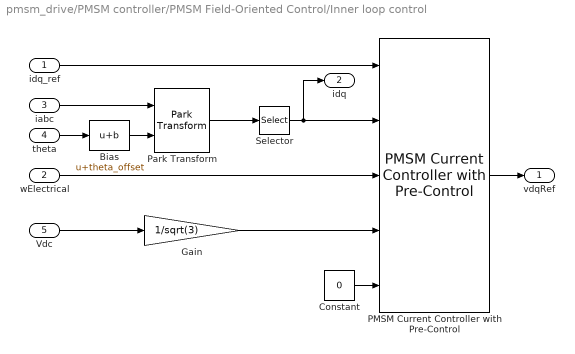
== system pmsm_drive/PMSM controller/PMSM Field-Oriented Control/Inner loop control ==
  idq_ref : Inport
  wElectrical : Inport  Port=2
  iabc : Inport  Port=3
  theta : Inport  Port=4
  Vdc : Inport  Port=5
  Bias : Bias  Bias=theta_offset
  Constant : Constant  Value=0  SampleTime=-1
  Gain : Gain  Gain=1/sqrt(3)
  PMSM Current Controller with Pre-Control : eePmsmCurrentController/PMSM Current Controller with Pre-Control  Kp_id=Kp_id  Ki_id=Ki_id  Kaw_id=Kaw_id  Kp_iq=Kp_iq  Ki_iq=Ki_iq  Kaw_iq=Kaw_iq  Ts=Tsc  Tsd=0.001  AxisPrio=Q-axis  ActZC=off  ActFF=on  idVect=idVect  iqVect=iqVect  LdMatrix=LdMatrix  LqMatrix=LqMatrix  psimMatrix=psimMatrix
      settings: SourceProductBaseCode=PS
  Park Transform : eeTransforms/Park Transform  AxisAlignment=Q-axis  PowerInvariant=off
  Selector : Selector  InputPortWidth=3  IndexOptions=Index vector (dialog)  Indices=[1 2]  OutputSizes=1
  vdqRef : Outport  VectorParamsAs1DForOutWhenUnconnected=off
  idq : Outport  Port=2  VectorParamsAs1DForOutWhenUnconnected=off
  wires:
  Bias/1 -> Park Transform/2
  PMSM Current Controller with Pre-Control/1 -> vdqRef/1
  Vdc/1 -> Gain/1
  wElectrical/1 -> PMSM Current Controller with Pre-Control/3
  theta/1 -> Bias/1
  iabc/1 -> Park Transform/1
  idq_ref/1 -> PMSM Current Controller with Pre-Control/1
  Park Transform/1 -> Selector/1
  Gain/1 -> PMSM Current Controller with Pre-Control/4
  Selector/1 -> idq/1, PMSM Current Controller with Pre-Control/2
  Constant/1 -> PMSM Current Controller with Pre-Control/5

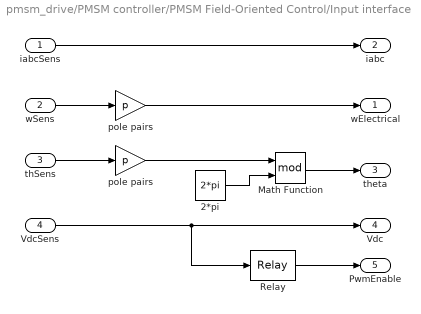
== system pmsm_drive/PMSM controller/PMSM Field-Oriented Control/Input interface ==
  iabcSens : Inport
  wSens : Inport  Port=2
  thSens : Inport  Port=3
  VdcSens : Inport  Port=4
  2*pi : Constant  Value=2*pi  SampleTime=Tsc
  Math Function : Math  Operator=mod  SignedPower=on  SaturateOnIntegerOverflow=on
  Relay : Relay  OnSwitchValue=Vdc_on  OffSwitchValue=0.5*Vdc_on
  pole pairs : Gain  Gain=p
  "pole pairs " : Gain  Gain=p
  wElectrical : Outport  VectorParamsAs1DForOutWhenUnconnected=off
  iabc : Outport  Port=2  VectorParamsAs1DForOutWhenUnconnected=off
  theta : Outport  Port=3  VectorParamsAs1DForOutWhenUnconnected=off
  Vdc : Outport  Port=4  VectorParamsAs1DForOutWhenUnconnected=off
  PwmEnable : Outport  Port=5  VectorParamsAs1DForOutWhenUnconnected=off
  wires:
  VdcSens/1 -> Vdc/1, Relay/1
  Relay/1 -> PwmEnable/1
  Math Function/1 -> theta/1
  2*pi/1 -> Math Function/2
  "pole pairs "/1 -> Math Function/1
  iabcSens/1 -> iabc/1
  wSens/1 -> pole pairs/1
  thSens/1 -> "pole pairs "/1
  pole pairs/1 -> wElectrical/1

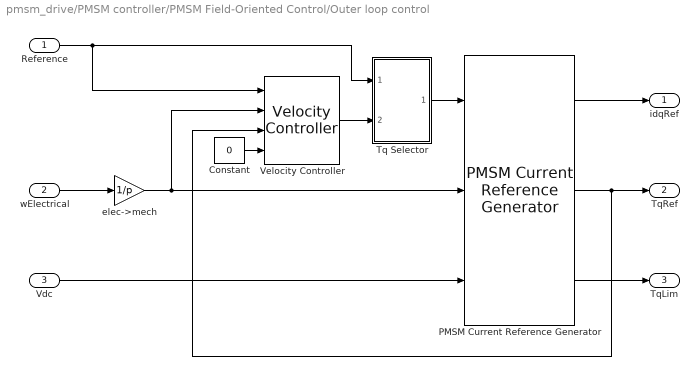
== system pmsm_drive/PMSM controller/PMSM Field-Oriented Control/Outer loop control ==
  Reference : Inport
  wElectrical : Inport  Port=2
  Vdc : Inport  Port=3
  Constant : Constant  Value=0  SampleTime=-1
  PMSM Current Reference Generator : eePmsmCurrentReferenceGen/PMSM Current Reference Generator  Vnom=Vnom  Pmax=Pmax  Tmax=Tmax  Ts=Tsc  RefType=Zero d-axis control  rpmVec=rpmVec  TqVec=TqVec  VdcVec=VdcVec  PWMMode=SPWM: sinusoidal PWM  ModFactor=ModFactor  idMatrix=idMatrix  iqMatrix=iqMatrix  p=p  psim=psim  Ld=Ld  Lq=Lq  Rs=Rs  RefExpEnable=0
      settings: SourceProductBaseCode=PS
  Tq Selector : Subsystem
  Velocity Controller : eeVelocityController/Velocity Controller  CtrlType=PI control  Kp_w=Kp_w  Ki_w=Ki_w  Kv_w=Kv_w  Kaw_w=Kaw_w  Ts=Tsc  Tsd=0.001  ActZC=off
      settings: SourceProductBaseCode=PS
  elec->mech : Gain  Gain=1/p
  idqRef : Outport  VectorParamsAs1DForOutWhenUnconnected=off
  TqRef : Outport  Port=2  VectorParamsAs1DForOutWhenUnconnected=off
  TqLim : Outport  Port=3  VectorParamsAs1DForOutWhenUnconnected=off
  wires:
  Velocity Controller/1 -> Tq Selector/2(TqRefUnsat)
  Tq Selector/1(TqRef) -> PMSM Current Reference Generator/1
  Constant/1 -> Velocity Controller/4
  elec->mech/1 -> Velocity Controller/2, PMSM Current Reference Generator/2
  PMSM Current Reference Generator/3 -> TqLim/1
  PMSM Current Reference Generator/2 -> TqRef/1, Velocity Controller/3
  PMSM Current Reference Generator/1 -> idqRef/1
  Vdc/1 -> PMSM Current Reference Generator/3
  wElectrical/1 -> elec->mech/1
  Reference/1 -> Tq Selector/1(Reference), Velocity Controller/1

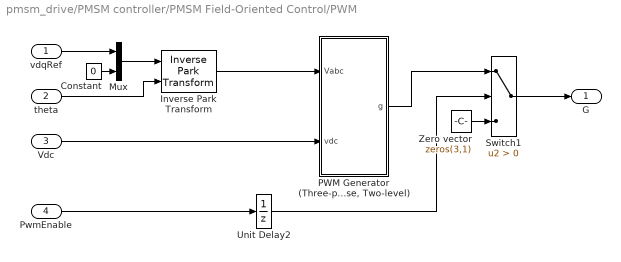
== system pmsm_drive/PMSM controller/PMSM Field-Oriented Control/PWM ==
  vdqRef : Inport
  theta : Inport  Port=2
  Vdc : Inport  Port=3
  PwmEnable : Inport  Port=4
  Constant : Constant  Value=0  SampleTime=Tsc
  Inverse Park Transform : eeTransforms/Inverse Park Transform  AxisAlignment=Q-axis  PowerInvariant=off
  Mux : Mux  Inputs=2
  "PWM Generator (Three-phase, Two-level)" : Subsystem  AncestorBlock=|  LoadFcn=ee_sli_rtmsupport( 'loadfcn', gcbh );  mask(PWM Generator (three-phase, two-level)){PWMMode=Continuous PWM (CPWM), CPWMMode=SPWM: sinusoidal PWM, DPWMMode=60 DPWM: 60 degree discontinuous PWM, SamplingMode=Natural, fsw=fsw, Ts=Ts}
      | eePwmGeneratorTwoLevel/PWM Generator
      | (Three-phase, Two-level)
      mask prompts: PWMMode "physmod:ee:library:comments:control:eePwmGeneratorTwoLevel:PWMMode_MP"; CPWMMode "physmod:ee:library:comments:control:eePwmGeneratorTwoLevel:ContinuousPWM_MP"; DPWMMode "physmod:ee:library:comments:control:eePwmGeneratorTwoLevel:DiscontinuousPWM_MP"; SamplingMode "physmod:ee:library:comments:control:eePwmGeneratorTwoLevel:SamplingMode_MP"; fsw "physmod:ee:library:comments:control:eePwmGeneratorTwoLevel:SwitchingFrequencyHz_MP"; Ts "physmod:ee:library:comments:control:eePwmGeneratorTwoLevel:SampleTimes_MP"
      mask help: physmod:ee:library:comments:control:eePwmGeneratorTwoLevel:PWMGeneratorthreephaseTwolevel_MD
      mask init:
      | Tsw = 1/fsw;
      | 
      | if fsw <= 0
      |     error(message('physmod:simscape:compiler:patterns:checks:GreaterThanZero',getString(message('physmod:ee:library:comments:control:eePwmGeneratorTwoLevel:SwitchingFrequencyHz_MP'))));
      | end
      | 
      | if Ts <= 0
      |     error(message('physmod:simscape:compiler:patterns:checks:GreaterThanZero',getString(message('physmod:ee:library:comments:control:eePwmGeneratorTwoLevel:SampleTimes_MP'))));
      | end
      | 
      | if Ts > 1/(10*fsw)
      |     error(message('physmod:simscape:compiler:patterns:checks:LessThanOrEqual',getString(message('physmod:ee:library:comments:control:eePwmGeneratorTwoLevel:SampleTimes_MP')),getString(message('physmod:ee:library:comments:control:eePwmGeneratorTwoLevel:inverseOf10TimesSwitchingFrequency_MP'))));
      | end
      | 
      | switch SamplingMode
      |     case 'Natural'
      |         RateTransitionOnInput = -1;
      |         GateGeneratorX0 = 0;
      |     case 'Asymmetric'
      |         RateTransitionOnInput = 0.5*Tsw;
      |         GateGeneratorX0 = 0.5/fsw;
      |     case 'Symmetric'
      |         RateTransitionOnInput = Tsw;
      |         GateGeneratorX0 = 0;
      | end
      | 
      | 
      | switch PWMMode
      |     case 'Continuous PWM (CPWM)'
      |         switch CPWMMode
      |             case 'SPWM: sinusoidal PWM'
      |                 PWM = 1;
      |             case 'SVM: space vector modulation'
      |                 PWM = 2;
      |         end
      |     case 'Discontinuous PWM (DPWM)'
      |         switch DPWMMode
      |             case '60 DPWM: 60 degree discontinuous PWM'
      |                 PWM = 3;
      |             case '60 DPWM (+30 degree shift): +30 degree shift from 60 DPWM'
      |                 PWM = 4;
      |             case '60 DPWM (-30 degree shift): -30 degree shift from 60 DPWM'
      |                 PWM = 5;
      |             case '30 DPWM: 30 degree discontinuous PWM'
      |                 PWM = 6;
      |             case '120 DPWM: positive dc component'
      |                 PWM = 7;
      |             case '120 DPWM: negative dc component'
      |                 PWM = 8;
      |         end
      | end
      settings: CopyFcn=ee_sli_rtmsupport( 'copyfcn', gcbh );  DeleteFcn=ee_sli_rtmsupport( 'deletefcn', gcbh );  ModelCloseFcn=ee_sli_rtmsupport( 'modelclosefcn', gcbh );  PreSaveFcn=%pe_sli_rtmsupport( 'presavefcn', gcbh );  PostSaveFcn=ee_sli_rtmsupport( 'postsavefcn', gcbh );  PreCopyFcn=ee_sli_rtmsupport( 'precopyfcn', gcbh );  OpenFcn=ee_sli_rtmsupport( 'openfcn', gcbh );  CloseFcn=ee_sli_rtmsupport( 'closefcn', gcbh );  PreDeleteFcn=ee_sli_rtmsupport( 'predeletefcn', gcbh );
      mask Help: web(nesl_help(gcbh))
      mask TypeOptions PWMMode: physmod:ee:library:comments:control:eePwmGeneratorTwoLevel:ContinuousPWMCPWM_PV | physmod:ee:library:comments:control:eePwmGeneratorTwoLevel:DiscontinuousPWMDPWM_PV
      mask Callback PWMMode:
      | switch get_param(gcb,'PWMMode')
      |     case 'Continuous PWM (CPWM)'
      |         set_param(gcb,'MaskVisibilities',{'on';'on';'off';'on';'on';'on'})
      |     case 'Discontinuous PWM (DPWM)'
      |         set_param(gcb,'MaskVisibilities',{'on';'off';'on';'on';'on';'on'})
      | end
      mask TypeOptions CPWMMode: physmod:ee:library:comments:control:eePwmGeneratorTwoLevel:SPWMSinusoidalPWM_PV | physmod:ee:library:comments:control:eePwmGeneratorTwoLevel:SVMSpaceVectorModulation_PV
      mask TypeOptions DPWMMode: physmod:ee:library:comments:control:eePwmGeneratorTwoLevel:x60DPWM60DegreeDiscontinuousPWM_PV | physmod:ee:library:comments:control:eePwmGeneratorTwoLevel:x60DPWM30DegreeShift30DegreeShiftFrom60DPWM_PV | physmod:ee:library:comments:control:eePwmGeneratorTwoLevel:x60DPWM0x2D30DegreeShift0x2D30DegreeShiftFrom60DPWM_PV | physmod:ee:library:comments:control:eePwmGeneratorTwoLevel:x30DPWM30DegreeDiscontinuousPWM_PV | physmod:ee:library:comments:control:eePwmGeneratorTwoLevel:x120DPWMPositiveDcComponent_PV | physmod:ee:library:comments:control:eePwmGeneratorTwoLevel:x120DPWMNegativeDcComponent_PV
      mask TypeOptions SamplingMode: physmod:ee:library:comments:control:eePwmGeneratorTwoLevel:Natural_PV | physmod:ee:library:comments:control:eePwmGeneratorTwoLevel:Asymmetric_PV | physmod:ee:library:comments:control:eePwmGeneratorTwoLevel:Symmetric_PV
      mask DialogControl ParameterGroupVar Prompt: physmod:ee:library:comments:control:eePwmGeneratorTwoLevel:tab_Parameters
      mask DialogControl PWMMode Prompt: PWM mode
      mask DialogControl CPWMMode Prompt: Continuous PWM
      mask DialogControl DPWMMode Prompt: Discontinuous PWM
      mask DialogControl SamplingMode Prompt: Sampling mode
      mask DialogControl fsw Prompt: Switching frequency (Hz)
      mask DialogControl Ts Prompt: Sample time (s)
  Switch1 : Switch  Criteria=u2 > Threshold
  Unit Delay2 : UnitDelay  SampleTime=Tsc  HasFrameUpgradeWarning=on
  Zero vector : Constant  Value=zeros(3,1)  SampleTime=Ts
  G : Outport  VectorParamsAs1DForOutWhenUnconnected=off
  wires:
  Unit Delay2/1 -> Switch1/2
  Vdc/1 -> "PWM Generator (Three-phase, Two-level)"/2(vdc)
  Inverse Park Transform/1 -> "PWM Generator (Three-phase, Two-level)"/1(Vabc)
  Switch1/1 -> G/1
  Zero vector/1 -> Switch1/3
  PwmEnable/1 -> Unit Delay2/1
  "PWM Generator (Three-phase, Two-level)"/1(g) -> Switch1/1
  Constant/1 -> Mux/2
  Mux/1 -> Inverse Park Transform/1
  vdqRef/1 -> Mux/1
  theta/1 -> Inverse Park Transform/2

== system pmsm_drive/PMSM controller/PMSM Field-Oriented Control/Outer loop control/Tq Selector ==
  Reference : Inport
  TqRefUnsat : Inport  Port=2
  Constant : Constant  Value=CtrlMode  SampleTime=Tsc
  Switch : Switch  Criteria=u2 > Threshold  Threshold=1.5
  TqRef : Outport  VectorParamsAs1DForOutWhenUnconnected=off
  wires:
  Switch/1 -> TqRef/1
  Constant/1 -> Switch/2
  TqRefUnsat/1 -> Switch/3
  Reference/1 -> Switch/1

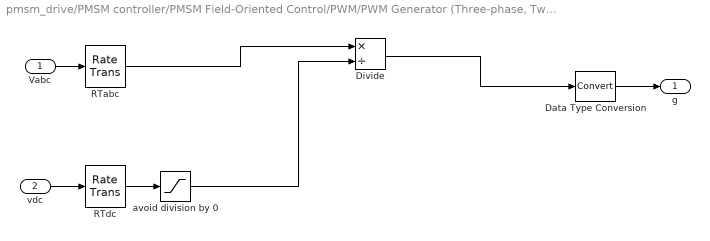
== system pmsm_drive/PMSM controller/PMSM Field-Oriented Control/PWM/PWM Generator (Three-phase, Two-level) ==
  Vabc : Inport
  vdc : Inport  Port=2
  Data Type Conversion : DataTypeConversion
  Divide : Product  Inputs=*/
  RTabc : RateTransition  OutPortSampleTime=RateTransitionOnInput
  RTdc : RateTransition  OutPortSampleTime=RateTransitionOnInput
  avoid division by 0 : Saturate  UpperLimit=inf  LowerLimit=eps
  g : Outport  VectorParamsAs1DForOutWhenUnconnected=off
  wires:
  avoid division by 0/1 -> Divide/2
  RTdc/1 -> avoid division by 0/1
  RTabc/1 -> Divide/1
  Data Type Conversion/1 -> g/1
  Divide/1 -> Data Type Conversion/1
  Vabc/1 -> RTabc/1
  vdc/1 -> RTdc/1
